simulink model "simlin"  (R2016a)
settings: Solver=VariableStepAuto  StartTime=0.0  StopTime=10.0  RelTol=1e-3
values from neighbouring files (symbols this model uses):
  Ac = eval(subs(Alin,[x1 x2 x3 x4 u],[xlin ulin]))    [linearizacia.m]    (also in linearnySM.mat = [0 0 0 0 1 0 0 0 0 -1.962 0 -58.86 ... (16 elements, 4x4)]; linearnySM2.mat = [0 0 0 0 1 0 0 0 0 -1.962 0 58.86 ... (16 elements, 4x4)]; sysd.mat = [0 0 0 0 1 0 0 0 0 -1.962 0 -58.86 ... (16 elements, 4x4)]; sysd2.mat = [0 0 0 0 1 0 0 0 0 -1.962 0 58.86 ... (16 elements, 4x4)])
  Bc = eval(subs(Blin,[x1 x2 x3 x4 u],[xlin ulin]))    [linearizacia.m]    (also in linearnySM.mat = [0 2.5 0 12.5]; linearnySM2.mat = [0 2.5 0 -12.5]; sysd.mat = [0 2.5 0 12.5]; sysd2.mat = [0 2.5 0 -12.5])
settings Model: Creator=gulan  LastModifiedBy=gulan

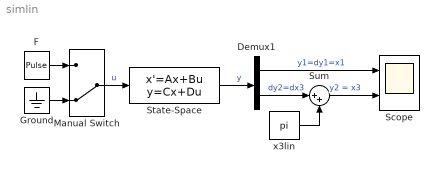
== system simlin ==
  " Scope" : Scope  NumInputPorts=2
  Demux1 : Demux  Outputs=2
  F : DiscretePulseGenerator  PulseType=Time based  Amplitude=-1  Period=10  PulseWidth=0.1  PhaseDelay=0.01
  Ground : Ground
  Manual Switch : ManualSwitch  CurrentSetting=0
  State-Space : StateSpace  A=Ac  B=Bc  C=eye(4)  D=zeros(4,1)  X0=[0;0;-pi/6;0]
  Sum : Sum  Inputs=|++
  x3lin : Constant  Value=pi
  wires:
  State-Space/1 -> Demux1/1  "y"
  F/1 -> Manual Switch/1
  Ground/1 -> Manual Switch/2
  Manual Switch/1 -> State-Space/1  "u"
  Demux1/1 -> " Scope"/1  "y1=dy1=x1"
  Demux1/2 -> Sum/1  "dy2=dx3"
  Sum/1 -> " Scope"/2  "y2 = x3"
  x3lin/1 -> Sum/2
